simulink model "Lire_Un_Enrouleur_RC4"  (R2024b)
settings: Solver=VariableStepAuto  StartTime=0.0  StopTime=10.0  RelTol=1e-3
settings Model: Creator=xpess  LastModifiedBy=xpess

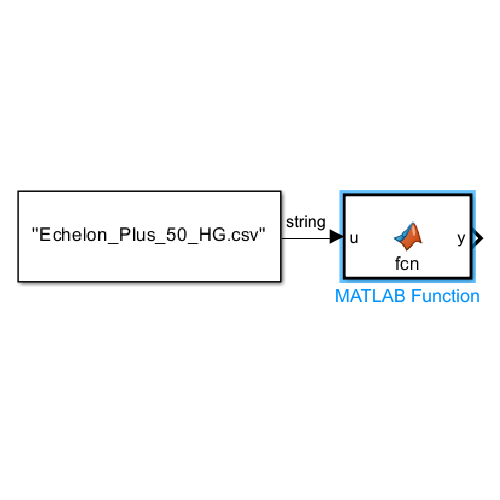
[thumbnail: Simulink's stored preview of the top-level diagram]
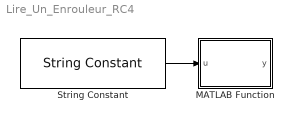
== system Lire_Un_Enrouleur_RC4 ==
  MATLAB Function : MATLAB Function  TreatAsAtomicUnit=on
  String Constant : StringConstant  String="\"Echelon_Plus_50_HG.csv\""
  wires:
  String Constant/1 -> MATLAB Function/1(u)

== matlab function Lire_Un_Enrouleur_RC4/MATLAB Function ==
  data: u input; y output
function y = fcn(u)

filename = u;
%%%%%
%function ts = parseMeasurementFile(filename)
    % Ouvre le fichier CSV
    fid = fopen(filename, 'r');

    % Vérifie si le fichier a été ouvert correctement
    if fid == -1
        error('Impossible d''ouvrir le fichier.');
    end

    % Lit la 8ème ligne pour obtenir le nombre de lignes de mesures et la période
    for i = 1:7
        fgetl(fid); % Saute les 7 premières lignes
    end
    line8 = fgetl(fid);

    % Extrait le nombre de lignes de mesures et la période en utilisant sscanf
    numMeasurements = sscanf(line8, '%d', 1);
    period = sscanf(fliplr(line8), '%d', 1);

    % Saute les lignes jusqu'à la 17ème ligne
    for i = 1:8
        fgetl(fid); % Saute les 8 lignes suivantes
    end

    % Initialise les matrices pour stocker les données
    data = zeros(numMeasurements, 7);

    % Lit les données ligne par ligne
    for i = 1:numMeasurements
        line = fgetl(fid);
        values = sscanf(line, '%f;%f;%f;%f;%f;%f;%f')';
        data(i, :) = values;
    end

    fclose(fid);

    % Extrait les colonnes nécessaires
    time = data(:, 2) / 1000; % Convertit le temps en secondes
    positionSetpoint = data(:, 4);
    positionMeasurement = data(:, 5);
    currentSetpoint = data(:, 6);
    currentMeasurement = data(:, 7);

    % Crée une série temporelle pour chaque mesure
    tsPositionSetpoint = timeseries(positionSetpoint, time, 'Name', 'PositionSetpoint');
    tsPositionMeasurement = timeseries(positionMeasurement, time, 'Name', 'PositionMeasurement');
    tsCurrentSetpoint = timeseries(currentSetpoint, time, 'Name', 'CurrentSetpoint');
    tsCurrentMeasurement = timeseries(currentMeasurement, time, 'Name', 'CurrentMeasurement');

    % Combine les séries temporelles dans une structure
    ts.PositionSetpoint = tsPositionSetpoint;
    ts.PositionMeasurement = tsPositionMeasurement;
    ts.CurrentSetpoint = tsCurrentSetpoint;
    ts.CurrentMeasurement = tsCurrentMeasurement;
%end




%%%%%%
y = ts;
